simulink model "thrusterMODEL"  (R2018a)
settings: Solver=VariableStepAuto  StartTime=0.0  StopTime=10.0  RelTol=1e-3
settings Model: Creator=varunpwr  LastModifiedBy=varunpwr

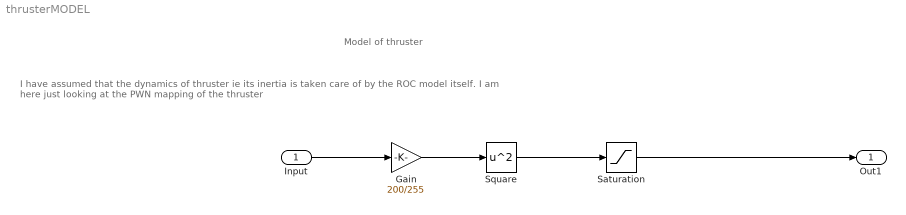
== system thrusterMODEL ==
  note: I have assumed that the dynamics of thruster ie its inertia is taken care of by the ROC model itself. I am here just looking at the PWN mapping of the thruster
  note: Model of thruster
  Input : Inport
  Gain : Gain  Gain=200/255
  Saturation : Saturate  UpperLimit=200  LowerLimit=-200
  Square : Math  Operator=square  SaturateOnIntegerOverflow=on
  Out1 : Outport
  wires:
  Gain/1 -> Square/1
  Input/1 -> Gain/1
  Square/1 -> Saturation/1
  Saturation/1 -> Out1/1
